simulink model "Ex2s"  (R2025a)
settings: Solver=VariableStepAuto  StartTime=0.0  StopTime=10.0  RelTol=1e-3
values from neighbouring files (symbols this model uses):
  sys2 = ss(A,B,C,D)    [Ex1.m]

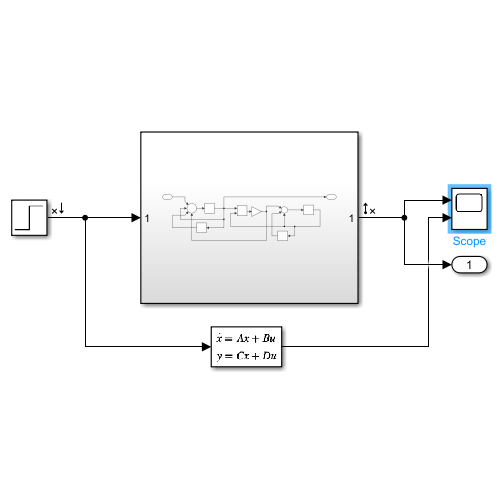
[thumbnail: Simulink's stored preview of the top-level diagram]
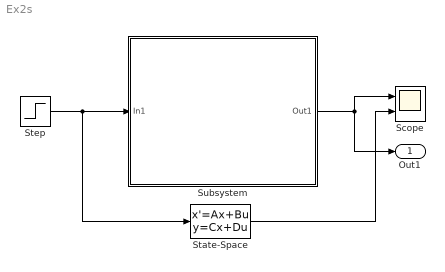
== system Ex2s ==
  Scope : Scope  NumInputPorts=2
      settings: ActiveDisplayYMinimum=-0.20225424726196597  ActiveDisplayYMaximum=1.8202882253576942
  State-Space : StateSpace  A=sys2.A  B=sys2.B  C=sys2.C  D=sys2.D  InitialCondition=0
  Step : Step  SampleTime=0
  Subsystem : Subsystem
  Out1 : Outport
  wires:
  Step/1 -> State-Space/1, Subsystem/1(In1)
  Subsystem/1(Out1) -> Out1/1, Scope/1
  State-Space/1 -> Scope/2

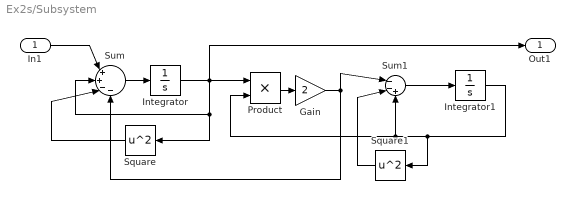
== system Ex2s/Subsystem ==
  In1 : Inport
  Gain : Gain  Gain=2
  Integrator : Integrator
  Integrator1 : Integrator
  Product : Product
  Square : Math  Operator=square
  Square1 : Math  Operator=square
  Sum : Sum  Inputs=|++--
  Sum1 : Sum  Inputs=|--+
  Out1 : Outport
  wires:
  In1/1 -> Sum/1
  Sum/1 -> Integrator/1
  Integrator/1 -> Out1/1, Product/1, Square/1, Sum/2
  Square/1 -> Sum/3
  Product/1 -> Gain/1
  Gain/1 -> Sum1/1, Sum/4
  Sum1/1 -> Integrator1/1
  Integrator1/1 -> Square1/1, Sum1/3, Product/2
  Square1/1 -> Sum1/2
